simulink model "CCS_1"  (R2019b)
settings: Solver=ode4  StartTime=0.0  StopTime=1000  FixedStep=0.5  RelTol=1e-3
settings Model: Creator=Administrator  LastModifiedBy=Administrator

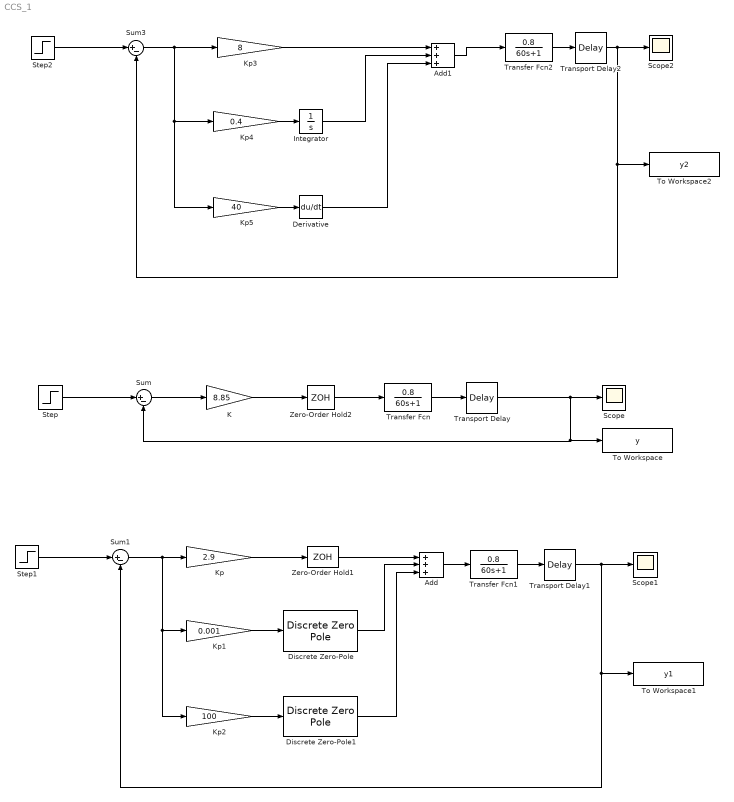
== system CCS_1 ==
  Add : Sum  Inputs=+++
  Add1 : Sum  Inputs=+++
  Derivative : Derivative
  Discrete Zero-Pole : DiscreteZeroPole  Zeros=[-1]  Poles=[1]  Gain=7.5  SampleTime=-1
  Discrete Zero-Pole1 : DiscreteZeroPole  Poles=[0]  Gain=0.0667  SampleTime=-1
  Integrator : Integrator
  K : Gain  Gain=8.85
  Kp : Gain  Gain=2.9
  Kp1 : Gain  Gain=0.001
  Kp2 : Gain  Gain=100
  Kp3 : Gain  Gain=8
  Kp4 : Gain  Gain=0.4
  Kp5 : Gain  Gain=40
  Scope : Scope
  Scope1 : Scope
  Scope2 : Scope
  Step : Step  Time=0  SampleTime=0
  Step1 : Step  Time=0  SampleTime=0
  Step2 : Step  Time=0  SampleTime=0
  Sum : Sum  Inputs=|+-
  Sum1 : Sum  Inputs=|+-
  Sum3 : Sum  Inputs=|+-
  To Workspace : ToWorkspace  VariableName=y  SaveFormat=Timeseries  SampleTime=-1
  To Workspace1 : ToWorkspace  VariableName=y1  SaveFormat=Timeseries  SampleTime=-1
  To Workspace2 : ToWorkspace  VariableName=y2  SaveFormat=Timeseries  SampleTime=-1
  Transfer Fcn : TransferFcn  Numerator=[0.8]  Denominator=[60 1]
  Transfer Fcn1 : TransferFcn  Numerator=[0.8]  Denominator=[60 1]
  Transfer Fcn2 : TransferFcn  Numerator=[0.8]  Denominator=[60 1]
  Transport Delay : TransportDelay  DelayTime=10
  Transport Delay1 : TransportDelay  DelayTime=60
  Transport Delay2 : TransportDelay  DelayTime=10
  Zero-Order Hold1 : ZeroOrderHold  SampleTime=15
  Zero-Order Hold2 : ZeroOrderHold  SampleTime=15
  wires:
  Step/1 -> Sum/1
  Sum/1 -> K/1
  Transfer Fcn/1 -> Transport Delay/1
  Transport Delay/1 -> To Workspace/1, Sum/2, Scope/1
  Transport Delay1/1 -> Scope1/1, To Workspace1/1, Sum1/2
  Step1/1 -> Sum1/1
  Sum1/1 -> Kp2/1, Kp1/1, Kp/1
  Transfer Fcn1/1 -> Transport Delay1/1
  Kp/1 -> Zero-Order Hold1/1
  Kp1/1 -> Discrete Zero-Pole/1
  Kp2/1 -> Discrete Zero-Pole1/1
  Transport Delay2/1 -> To Workspace2/1, Sum3/2, Scope2/1
  Transfer Fcn2/1 -> Transport Delay2/1
  Step2/1 -> Sum3/1
  K/1 -> Zero-Order Hold2/1
  Zero-Order Hold2/1 -> Transfer Fcn/1
  Discrete Zero-Pole/1 -> Add/2
  Discrete Zero-Pole1/1 -> Add/3
  Zero-Order Hold1/1 -> Add/1
  Add/1 -> Transfer Fcn1/1
  Kp5/1 -> Derivative/1
  Kp4/1 -> Integrator/1
  Integrator/1 -> Add1/2
  Derivative/1 -> Add1/3
  Sum3/1 -> Kp5/1, Kp4/1, Kp3/1
  Add1/1 -> Transfer Fcn2/1
  Kp3/1 -> Add1/1
